simulink model "Question6_model"  (R2021a)
settings: Solver=VariableStepAuto  StartTime=0.0  StopTime=10.0  RelTol=1e-3
values from neighbouring files (symbols this model uses):
  A = [-1.7 -0.25 0; 23 -30 20; 0 -450 -740]    [Question6.m]
  B = [5 0; -44 0; 0 -830]    [Question6.m]
  Cd = [1 0 0;0 1 0;0 0 1]    [Question6.m]
settings Model: Creator=Arunava  LastModifiedBy=l_w_h

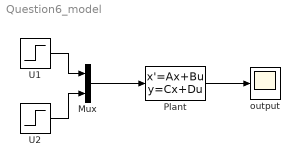
== system Question6_model ==
  Mux : Mux  Inputs=2
  Plant : StateSpace  A=A  B=B  C=Cd  D=[0 0;0 0;0 0]  InitialCondition=0
  U1 : Step  Time=0  After=15.5813  SampleTime=0
  U2 : Step  Time=0  After=-410.7783  SampleTime=0
  output : Scope
  wires:
  U1/1 -> Mux/1
  U2/1 -> Mux/2
  Mux/1 -> Plant/1
  Plant/1 -> output/1
